simulink model "demo_simulink_2022b"  (R2023a)
settings: Solver=ode23t  StartTime=0.0  StopTime=20  RelTol=1e-3
values from neighbouring files (symbols this model uses):
  alpha = 0.1    [constants.m]
  ALPHA = 75    [constants.m]
  BETA = 0.8    [constants.m]
  GAMMA = 0.5    [constants.m]
  k = 10    [constants.m]
  m = 1    [constants.m]
  N_BOUNCES = 10    [constants.m]
  V = 10    [constants.m]
  v_0 = 20    [constants.m]
  x_0 = 1    [constants.m]
undefined symbols (not defined in the file or in its folder): A, B, K_I, K_P, T1, T2
libraries: simulink x5, dspswit3 x1
settings Model: Creator=Артём  LastModifiedBy=ycheb

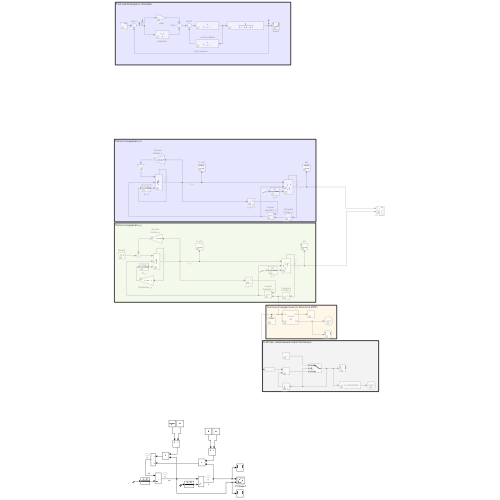
[thumbnail: Simulink's stored preview of the top-level diagram]
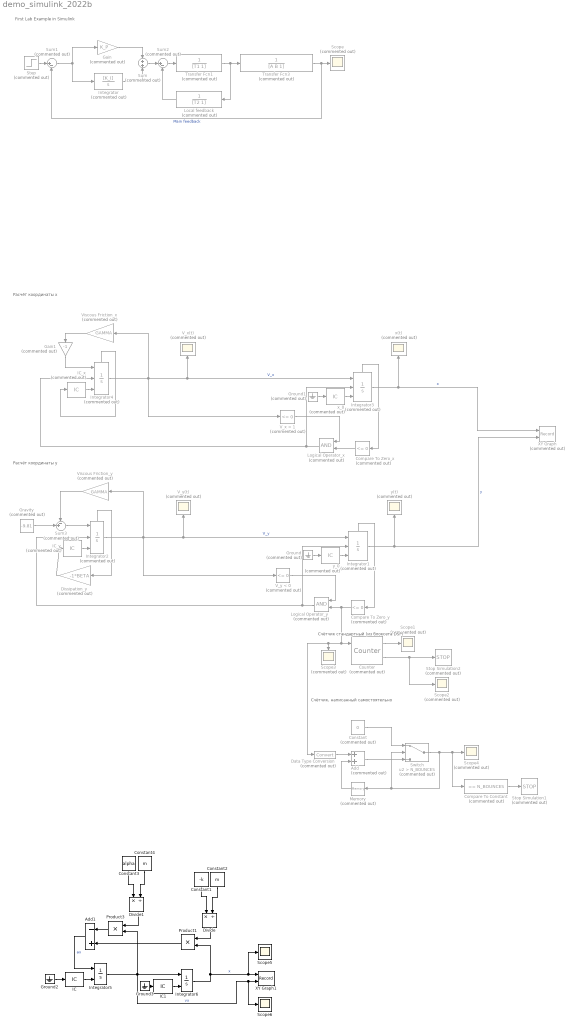
== system demo_simulink_2022b ==
  note: Счётчик, написанный самостоятельно
  note: Счётчик стандартный (из блоксета DSP)
  note: Расчёт координаты y
  note: Расчёт координаты x
  note: First Lab Example in Simulink
  Add : Sum  Commented=on
  Add1 : Sum  Inputs=-+
  Compare To Constant : simulink/Logic and Bit Operations/Compare To Constant  Commented=on  relop===  const=N_BOUNCES  OutDataTypeStr=boolean
  Compare To Zero_x : simulink/Logic and Bit Operations/Compare To Zero  Commented=on  relop=<=  OutDataTypeStr=boolean
  Compare To Zero_y : simulink/Logic and Bit Operations/Compare To Zero  Commented=on  relop=<=  OutDataTypeStr=boolean
  Constant : Constant  Commented=on  Value=0
  Constant1 : Constant  Value=-k
  Constant2 : Constant  Value=m
  Constant3 : Constant  Value=alpha
  Constant4 : Constant  Value=m
  Counter : dspswit3/Counter  Commented=on  Direction=Up  CountEvent=Rising edge  CounterSize=User defined  MaxCount=255  InitialCount=0  Output=Count and Hit  HitValue=N_BOUNCES  ResetInput=on  SamplesPerFrame=1  Ts=1  CntDtype=double  HitDtype=Boolean
  Data Type Conversion : DataTypeConversion  Commented=on  SaturateOnIntegerOverflow=off  RndMeth=Floor
  Dissipation_y : Gain  Commented=on  Gain=-1*BETA
  Divide : Product  Inputs=*/
  Divide1 : Product  Inputs=*/
  Gain : Gain  Commented=on  Gain=K_P
  Gain1 : Gain  Commented=on  Gain=-1
  Gravity : Constant  Commented=on  Value=-9.81
  Ground : Ground  Commented=on
  Ground1 : Ground  Commented=on
  Ground2 : Ground
  Ground3 : Ground
  IC : InitialCondition  Value=v_0
  IC1 : InitialCondition  Value=x_0
  IC_x : InitialCondition  Commented=on  Value=V * cos(ALPHA * pi / 180)
  IC_y : InitialCondition  Commented=on  Value=V * sin(ALPHA * pi / 180)
  Integrator : TransferFcn  Commented=on  Numerator=[K_I]  Denominator=[1 0]
  Integrator1 : Integrator  Commented=on  ExternalReset=rising  InitialConditionSource=external  LimitOutput=on  LowerSaturationLimit=0  ShowStatePort=on
  Integrator2 : Integrator  Commented=on  ExternalReset=rising  InitialConditionSource=external  ShowStatePort=on
  Integrator3 : Integrator  Commented=on  ExternalReset=rising  InitialConditionSource=external  LimitOutput=on  LowerSaturationLimit=0  ShowStatePort=on
  Integrator4 : Integrator  Commented=on  ExternalReset=rising  InitialConditionSource=external  ShowStatePort=on
  Integrator5 : Integrator  InitialConditionSource=external
  Integrator6 : Integrator  InitialConditionSource=external
  Local feedback : TransferFcn  Commented=on  Denominator=[T2 1]
  Logical Operator_x : Logic  Commented=on  AllPortsSameDT=off  OutDataTypeStr=boolean
  Logical Operator_y : Logic  Commented=on  AllPortsSameDT=off  OutDataTypeStr=boolean
  Memory : Memory  Commented=on  InitialCondition=-1
  Product1 : Product
  Product3 : Product
  Scope{,1..4} (5 alike) : Scope  Commented=on
  Scope5 : Scope
  Scope6 : Scope
  Step : Step  Commented=on  Time=0.1  SampleTime=0
  Stop Simulation1 : Stop  Commented=on
  Stop Simulation2 : Stop  Commented=on
  Sum : Sum  Commented=on  Inputs=+|+
  Sum1 : Sum  Commented=on  Inputs=|+-
  Sum2 : Sum  Commented=on  Inputs=|+-
  Sum3 : Sum  Commented=on  Inputs=-+|
  Switch : Switch  Commented=on  Criteria=u2 > Threshold  Threshold=N_BOUNCES  SaturateOnIntegerOverflow=off  InputSameDT=off
  Transfer Fcn1 : TransferFcn  Commented=on  Denominator=[T1 1]
  Transfer Fcn3 : TransferFcn  Commented=on  Denominator=[A B 1]
  V_x < 1 : simulink/Logic and Bit Operations/Compare To Zero  Commented=on  relop=<=  OutDataTypeStr=boolean
  V_x(t) : Scope  Commented=on
  V_y < 0 : simulink/Logic and Bit Operations/Compare To Zero  Commented=on  relop=<=  OutDataTypeStr=boolean
  V_y(t) : Scope  Commented=on
  Viscous Friction_x : Gain  Commented=on  Gain=GAMMA
  Viscous Friction_y : Gain  Commented=on  Gain=GAMMA
  XY Graph : Record  Commented=on  FileSettingsInternal="{\"entries\":[{\"content\":{\"excelSettings\":{\"content\":{},\"type\":\"Streamout.ExcelSettings\"}},\"type\":\"Streamout.FileSettingStorage\",\"uuid\":\"\"}],\"packageUris\":[\"http:\\/\\/schema.mathworks.com\\/mf0\\/streamout_blocks\\/R2020a\"],\"version\":\"1.0\"}"  Layout=[1 1]  SignalsInternal="{\"entries\":[{\"content\":{},\"type\":\"RecordBlkView.InputSignals\",\"uuid\":\"\"}],\"packageUris\":[\"http:\\/\\/schema.mathworks.com\\/mf0\\/streamout_blocks\\/R2020a\"],\"version\":\"1.0\"}"  VisualizationBindings="{\"xyplotplugin\":{\"info\":[{\"series\":[],\"subplotID\":1}]}}"  CompatibilityTag=XY
  XY Graph1 : Record  FileSettingsInternal="{\"entries\":[{\"content\":{\"excelSettings\":{\"content\":{},\"type\":\"Streamout.ExcelSettings\"}},\"type\":\"Streamout.FileSettingStorage\",\"uuid\":\"\"}],\"packageUris\":[\"http:\\/\\/schema.mathworks.com\\/mf0\\/streamout_blocks\\/R2020a\"],\"version\":\"1.0\"}"  Layout=[1 1]  SignalsInternal="{\"entries\":[{\"content\":{\"signals\":[{\"content\":{\"blockPath\":[],\"dimensions\":[1],\"domain\":\"\",\"lineColor\":\"#a2142f\",\"plots\":[1],\"port\":1,\"sid\":[\"\"],\"signalID\":240,\"signalName\":\"x\"},\"type\":\"RecordBlkView.Signal\",\"uuid\":\"\"},{\"content\":{\"blockPath\":[],\"dimensions\":[1],\"domain\":\"\",\"lineColor\":\"#139fff\",\"plots\":[1],\"port\":2,\"sid\":[\"\"],\"signalID\":244,\"signalName\":\"vx\"},\"type\":\"RecordBlkView.Signal\",\"uuid\":\"\"}]},\"type\":\"RecordBlkView.InputSignals\",\"uuid\":\"\"}],\"packageUris\":[\"http:\\/\\/schema.mathworks.com\\/mf0\\/streamout_blocks\\/R2020a\"],\"version\":\"1.0\"}"  VisualizationBindings="{\"xyplotplugin\":{\"info\":[{\"series\":[{\"bindingParametersList\":[{\"parameter\":\"X-Axis\",\"signalID\":240,\"signalName\":\"x\"},{\"parameter\":\"Y-Axis\",\"signalID\":244,\"signalName\":\"vx\"}],\"seriesID\":28048}],\"subplotID\":1}]}}"  CompatibilityTag=XY
  x(t) : Scope  Commented=on
  x_0 : InitialCondition  Commented=on  Value=0
  y(t) : Scope  Commented=on
  y_0 : InitialCondition  Commented=on  Value=0
  wires:
  Integrator/1 -> Sum/2
  Sum1/1 -> Gain/1, Integrator/1
  Sum/1 -> Sum2/1
  Sum2/1 -> Transfer Fcn1/1
  Local feedback/1 -> Sum2/2
  Transfer Fcn1/1 -> Local feedback/1, Transfer Fcn3/1
  Transfer Fcn3/1 -> Sum1/2, Scope/1  "Main feedback"
  Step/1 -> Sum1/1
  Gain/1 -> Sum/1
  Integrator2/1 -> Viscous Friction_y/1, V_y < 0/1, V_y(t)/1, Integrator1/1  "V_y"
  Integrator1/1 -> XY Graph/2, y(t)/1  "y"
  IC_y/1 -> Integrator2/3
  Logical Operator_y/1 -> Integrator2/2, Integrator1/2
  y_0/1 -> Integrator1/3
  Dissipation_y/1 -> IC_y/1
  Gravity/1 -> Sum3/2
  Ground/1 -> y_0/1
  V_y < 0/1 -> Logical Operator_y/1
  Integrator2/State -> Dissipation_y/1
  Integrator1/State -> Compare To Zero_y/1
  Viscous Friction_y/1 -> Sum3/1
  Sum3/1 -> Integrator2/1
  Gain1/1 -> Integrator4/1
  x_0/1 -> Integrator3/3
  V_x < 1/1 -> Logical Operator_x/1
  Integrator3/State -> Compare To Zero_x/1
  Integrator3/1 -> XY Graph/1, x(t)/1  "x"
  Compare To Zero_x/1 -> Logical Operator_x/2
  Viscous Friction_x/1 -> Gain1/1
  Ground1/1 -> x_0/1
  IC_x/1 -> Integrator4/3
  Integrator4/State -> IC_x/1
  Logical Operator_x/1 -> Integrator4/2, Integrator3/2
  Integrator4/1 -> Viscous Friction_x/1, V_x < 1/1, V_x(t)/1, Integrator3/1  "V_x"
  Counter/2 -> Stop Simulation2/1, Scope2/1
  Counter/1 -> Scope1/1
  Memory/1 -> Add/2
  Add/1 -> Switch/3
  Switch/1 -> Compare To Constant/1, Scope4/1, Switch/2, Memory/1
  Constant/1 -> Switch/1
  Data Type Conversion/1 -> Add/1
  Compare To Constant/1 -> Stop Simulation1/1
  Compare To Zero_y/1 -> Data Type Conversion/1, Scope3/1, Counter/1, Logical Operator_y/2
  Constant1/1 -> Divide/1
  Constant2/1 -> Divide/2
  Divide/1 -> Product1/1
  Integrator6/1 -> XY Graph1/1, Scope5/1, Product1/2  "x"
  Divide1/1 -> Product3/1
  Integrator5/1 -> Product3/2, XY Graph1/2, Scope6/1, Integrator6/1  "vx"
  Constant3/1 -> Divide1/1
  Constant4/1 -> Divide1/2
  Product3/1 -> Add1/1
  Product1/1 -> Add1/2
  Add1/1 -> Integrator5/1  "ax"
  IC/1 -> Integrator5/2
  Ground2/1 -> IC/1
  Ground3/1 -> IC1/1
  IC1/1 -> Integrator6/2
